simulink model "VOO"  (R2022a)
settings: Solver=FixedStepAuto  StartTime=0.0  StopTime=10.0  FixedStep=1e-3  RelTol=1e-3  EnableMultiTasking=on
undefined symbols (not defined in the file): D10, D11, D12, D13, D2, D3, D4, D5, D6, D7, D8, D9, PTA0, PTA1, PTA2, PTB23, PTB9, PTC2, PTC3, PTC4, PTD0, PTD1, PTD2, PTD3
libraries: frdmk64flib x13
settings Model: ExtModeTrigDuration=5  Creator=12791  LastModifiedBy=12791
settings OptimizationCC: EnhancedBackFolding=on  PassReuseOutputArgsAs=Individual arguments  ZeroExternalMemoryAtStartup=off  ZeroInternalMemoryAtStartup=off  MaxStackSize=64  OptimizeBlockOrder=speed  DifferentSizesBufferReuse=on  OptimizationCustomize=off  EfficientTunableParamExpr=on
settings DebuggingCC: ParameterTunabilityLossMsg=error
settings HardwareCC: ProdBitPerPointer=32  ProdBitPerSizeT=32  ProdBitPerPtrDiffT=32  ProdLargestAtomicInteger=Long  ProdLargestAtomicFloat=Double  ProdWordSize=32  ProdHWDeviceType=ARM Compatible->ARM Cortex
settings SFSimCC: MATLABDynamicMemAlloc=off
settings RTWCC: SystemTargetFile=ert.tlc  HardwareBoard=NXP FRDM-K64F  TLCOptions="-aInlineSetEventsForThisBaseRateFcn=TLC_FALSE -aSuppressMultiTaskScheduler=TLC_FALSE  -aRateBasedStepFcn=0"  TemplateMakefile=ert_default_tmf  Toolchain=GNU Tools for ARM Embedded Processors
settings CodeAppCC: ForceParamTrailComments=on  IgnoreCustomStorageClasses=off  OperatorAnnotations=on  SimulinkDataObjDesc=on  SFDataObjDesc=on  InsertBlockDesc=on
settings ERTTargetCC: ExtModeTransport=4  ExtModeMexFile=sendToCommService

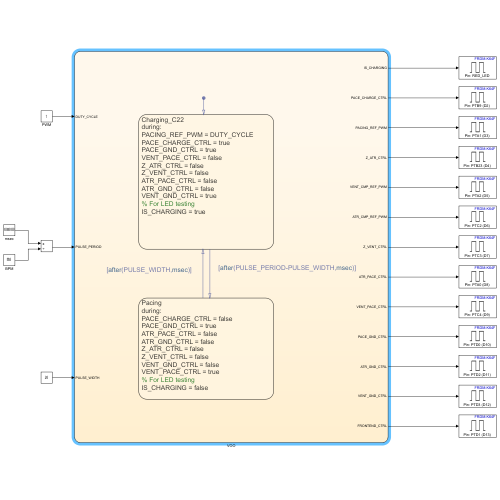
[thumbnail: Simulink's stored preview of the top-level diagram]
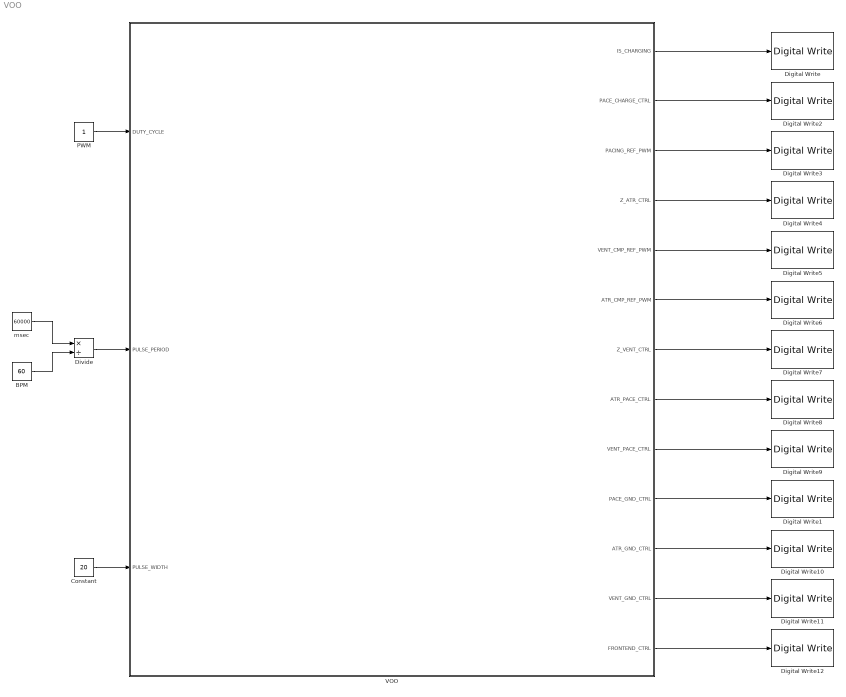
== system VOO ==
  BPM : Constant  Value=60
  Constant : Constant  Value=20
  Digital Write : frdmk64flib/Digital Write  Whichpin=RED_LED
  Digital Write1 : frdmk64flib/Digital Write  Whichpin=PTD0 (D10)
  Digital Write10 : frdmk64flib/Digital Write  Whichpin=PTD2 (D11)
  Digital Write11 : frdmk64flib/Digital Write  Whichpin=PTD3 (D12)
  Digital Write12 : frdmk64flib/Digital Write  Whichpin=PTD1 (D13)
  Digital Write2 : frdmk64flib/Digital Write  Whichpin=PTB9 (D2)
  Digital Write3 : frdmk64flib/Digital Write  Whichpin=PTA1 (D3)
  Digital Write4 : frdmk64flib/Digital Write  Whichpin=PTB23 (D4)
  Digital Write5 : frdmk64flib/Digital Write  Whichpin=PTA2 (D5)
  Digital Write6 : frdmk64flib/Digital Write  Whichpin=PTC2 (D6)
  Digital Write7 : frdmk64flib/Digital Write  Whichpin=PTC3 (D7)
  Digital Write8 : frdmk64flib/Digital Write  Whichpin=PTA0 (D8)
  Digital Write9 : frdmk64flib/Digital Write  Whichpin=PTC4 (D9)
  Divide : Product  Inputs=*/
  PWM : Constant
  VOO : Stateflow chart  TreatAsAtomicUnit=on
  msec : Constant  Value=60000
  wires:
  VOO/2(PACE_CHARGE_CTRL) -> Digital Write2/1
  VOO/3(PACING_REF_PWM) -> Digital Write3/1
  VOO/4(Z_ATR_CTRL) -> Digital Write4/1
  VOO/5(VENT_CMP_REF_PWM) -> Digital Write5/1
  VOO/6(ATR_CMP_REF_PWM) -> Digital Write6/1
  VOO/7(Z_VENT_CTRL) -> Digital Write7/1
  VOO/8(ATR_PACE_CTRL) -> Digital Write8/1
  VOO/9(VENT_PACE_CTRL) -> Digital Write9/1
  VOO/10(PACE_GND_CTRL) -> Digital Write1/1
  VOO/11(ATR_GND_CTRL) -> Digital Write10/1
  VOO/12(VENT_GND_CTRL) -> Digital Write11/1
  VOO/13(FRONTEND_CTRL) -> Digital Write12/1
  PWM/1 -> VOO/1(DUTY_CYCLE)
  Constant/1 -> VOO/3(PULSE_WIDTH)
  Divide/1 -> VOO/2(PULSE_PERIOD)
  msec/1 -> Divide/1
  BPM/1 -> Divide/2
  VOO/1(IS_CHARGING) -> Digital Write/1

== stateflow chart VOO/VOO ==
  state Charging_C22
    during:
    PACING_REF_PWM = DUTY_CYCLE
    PACE_CHARGE_CTRL = true
    PACE_GND_CTRL = true
    VENT_PACE_CTRL = false
    Z_ATR_CTRL = false
    Z_VENT_CTRL = false
    ATR_PACE_CTRL = false
    ATR_GND_CTRL = false
    VENT_GND_CTRL = true
    % For LED testing
    IS_CHARGING = true
  state Pacing
    during:
    PACE_CHARGE_CTRL = false
    PACE_GND_CTRL = true
    ATR_PACE_CTRL = false
    ATR_GND_CTRL = false
    Z_ATR_CTRL = false
    Z_VENT_CTRL = false
    VENT_GND_CTRL = false
    VENT_PACE_CTRL = true
    % For LED testing
    IS_CHARGING = false
  (default) -> Charging_C22
  Pacing -> Charging_C22 : [after(PULSE_WIDTH,msec)]
  Charging_C22 -> Pacing : [after(PULSE_PERIOD-PULSE_WIDTH,msec)]
  data: IS_CHARGING output; PACE_CHARGE_CTRL output; PACING_REF_PWM output; Z_ATR_CTRL output; VENT_CMP_REF_PWM output =false; ATR_CMP_REF_PWM output =false; Z_VENT_CTRL output; ATR_PACE_CTRL output; VENT_PACE_CTRL output; PACE_GND_CTRL output; ATR_GND_CTRL output; VENT_GND_CTRL output; FRONTEND_CTRL output =true; DUTY_CYCLE input; PULSE_PERIOD input; PULSE_WIDTH input
